simulink model "EvReferenceApplication"  (R2017b)
settings: Solver=ode23tb  StartTime=0  StopTime=600  RelTol=1e-3  EnableMultiTasking=on
InitFcn:
  | %open_system('EvReferenceApplication/Visualization/Performance and FE Scope');
undefined symbols (not defined in the file): ACC_Dgap_m, ACC_Kd, ACC_Ki, ACC_Kp, ACC_Nf, ACC_Tgap_s, BattChargeMax, UseAdaptiveCruiseControl_bool
libraries: autolibshared x2, autolibsharedcommon x1, simulink x1
settings Model: ModifiedByFormat=The MathWorks, Inc.  SimulationMode=accelerator  PauseTimes=23.46  Creator=The MathWorks, Inc.  LastModifiedBy=The MathWorks, Inc.
settings SolverCC: DecoupledContinuousIntegration=on
settings DataIOCC: DSMLogging=off
settings DebuggingCC: UnderspecifiedInitializationDetection=Classic  MergeDetectMultiDrivingBlocksExec=none  ModelReferenceExtraNoncontSigs=none
settings ModelReferenceCC: UpdateModelReferenceTargets=IfOutOfDate  EnableParallelModelReferenceBuilds=on  ModelReferenceMinAlgLoopOccurrences=on  PropagateSignalLabelsOutOfModel=off
settings CodeAppCC: StateflowObjectComments=on
settings GRTTargetCC: TargetLangStandard=C89/C90 (ANSI)
settings ConfigComp: CovMetricSettings=dsw  CovHtmlReporting=on  CovSaveCumulativeToWorkspaceVar=on  CovSaveSingleToWorkspaceVar=on  CovShowResultsExplorer=off  CovExternalEMLEnable=off

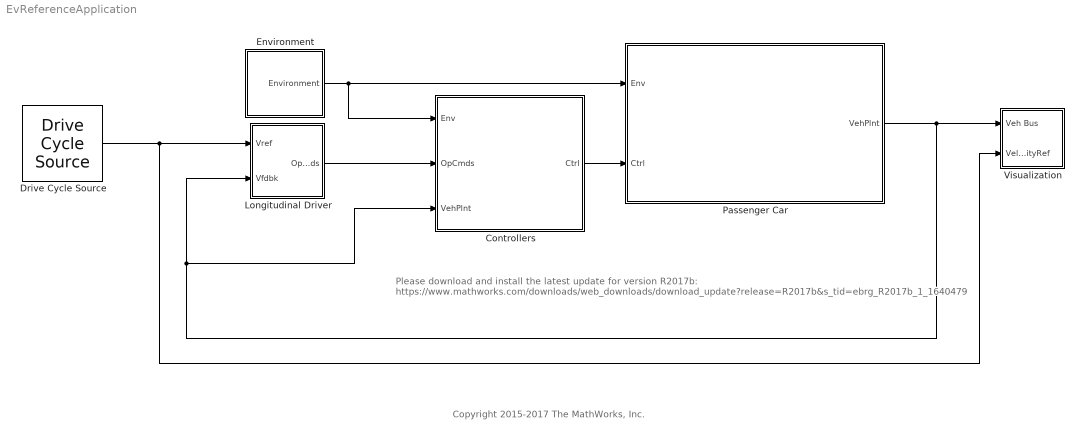
== system EvReferenceApplication ==
  note: Copyright 2015-2017 The MathWorks, Inc.
  note: Please download and install the latest update for version R2017b: https://www.mathworks.com/downloads/web_downloads/download_update?release=R2017b&s_tid=ebrg_R2017b_1_1640479
  Controllers : Subsystem
      mask Display: image('SystemControllers.png','center')
  Drive Cycle Source : autolibshared/Drive Cycle Source  cycleVar=US06  tfinal="600  seconds"  cycleRepeat=off  outAccPort=off  t_wot1=1  xdot_woto=0  xdot_wot1=26.8  t_wot2=30  xdot_wot2=0  t_wotend=40  srcUnit=m/s  outUnit=m/s  srcAccUnit=m/s/s  outAccUnit=m/s^2  dt=0
      settings: SourceProductName=Powertrain Blockset  SourceProductBaseCode=PW
  Environment : Subsystem
      mask Display: disp('Environment')
  Longitudinal Driver : Subsystem
      mask Display: image('LongitudinalDriver.png', 'center')
  Passenger Car : Subsystem
      mask Display: image('PassengerVehicle.png','center')
  Visualization : Subsystem
      mask Display: disp('Visualization')
  wires:
  Longitudinal Driver/1(OpCmds) -> Controllers/2(OpCmds)
  Drive Cycle Source/1 -> Longitudinal Driver/1(Vref), Visualization/2(VelocityRef)
  Environment/1(Environment) -> Controllers/1(Env), Passenger Car/1(Env)
  Controllers/1(Ctrl) -> Passenger Car/2(Ctrl)
  Passenger Car/1(VehPlnt) -> Controllers/3(VehPlnt), Longitudinal Driver/2(Vfdbk), Visualization/1(Veh Bus)

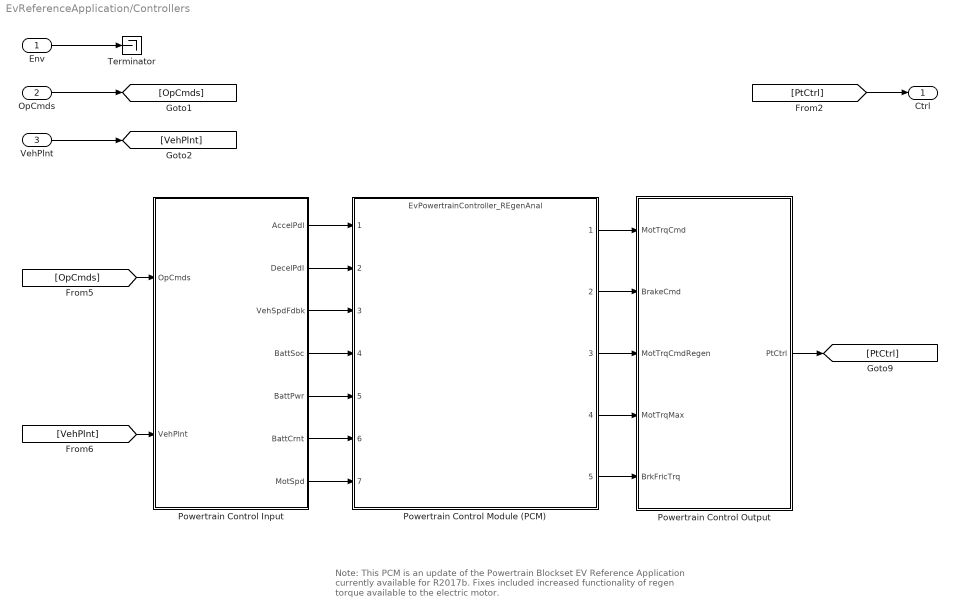
== system EvReferenceApplication/Controllers ==
  note: Note: This PCM is an update of the Powertrain Blockset EV Reference Application currently available for R2017b. Fixes included increased functionality of regen torque available to the electric motor.
  Env : Inport
  OpCmds : Inport  Port=2
  VehPlnt : Inport  Port=3
  Powertrain Control Input : Subsystem
  Powertrain Control Module (PCM) : ModelReference  ModelNameDialog=EvPowertrainController_REgenAnal.slx  SimulationMode=Normal  ModelReferenceVersion=1.420
  Powertrain Control Output : Subsystem
  Terminator : Terminator
  Ctrl : Outport
  wires:
  [PtCtrl] -> Ctrl/1
  Env/1 -> Terminator/1
  [OpCmds] -> Powertrain Control Input/1(OpCmds)
  Powertrain Control Output/1(PtCtrl) -> [PtCtrl]
  [VehPlnt] -> Powertrain Control Input/2(VehPlnt)
  VehPlnt/1 -> [VehPlnt]
  OpCmds/1 -> [OpCmds]
  Powertrain Control Input/4(BattSoc) -> Powertrain Control Module (PCM)/4
  Powertrain Control Input/3(VehSpdFdbk) -> Powertrain Control Module (PCM)/3
  Powertrain Control Input/2(DecelPdl) -> Powertrain Control Module (PCM)/2
  Powertrain Control Input/1(AccelPdl) -> Powertrain Control Module (PCM)/1
  Powertrain Control Input/5(BattPwr) -> Powertrain Control Module (PCM)/5
  Powertrain Control Input/6(BattCrnt) -> Powertrain Control Module (PCM)/6
  Powertrain Control Input/7(MotSpd) -> Powertrain Control Module (PCM)/7
  Powertrain Control Module (PCM)/1 -> Powertrain Control Output/1(MotTrqCmd)
  Powertrain Control Module (PCM)/2 -> Powertrain Control Output/2(BrakeCmd)
  Powertrain Control Module (PCM)/3 -> Powertrain Control Output/3(MotTrqCmdRegen)
  Powertrain Control Module (PCM)/4 -> Powertrain Control Output/4(MotTrqMax)
  Powertrain Control Module (PCM)/5 -> Powertrain Control Output/5(BrkFricTrq)

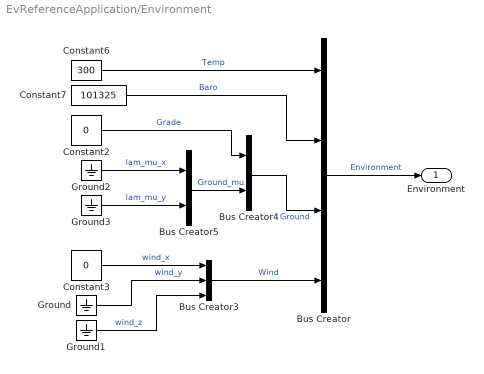
== system EvReferenceApplication/Environment ==
  Bus Creator : BusCreator  Inputs=4
  Bus Creator3 : BusCreator  Inputs=3
  Bus Creator4 : BusCreator  Inputs=2
  Bus Creator5 : BusCreator  Inputs=2
  Constant2 : Constant  Value=0
  Constant3 : Constant  Value=0
  Constant6 : Constant  Value=300
  Constant7 : Constant  Value=101325
  Ground{,1..3} (4 alike) : Ground
  Environment : Outport
  wires:
  Ground2/1 -> Bus Creator5/1  "lam_mu_x"
  Ground3/1 -> Bus Creator5/2  "lam_mu_y"
  Bus Creator5/1 -> Bus Creator4/2  "Ground_mu"
  Bus Creator4/1 -> Bus Creator/3  "Ground"
  Bus Creator3/1 -> Bus Creator/4  "Wind"
  Constant3/1 -> Bus Creator3/1  "wind_x"
  Ground/1 -> Bus Creator3/2  "wind_y"
  Ground1/1 -> Bus Creator3/3  "wind_z"
  Constant6/1 -> Bus Creator/1  "Temp"
  Constant2/1 -> Bus Creator4/1  "Grade"
  Bus Creator/1 -> Environment/1  "Environment"
  Constant7/1 -> Bus Creator/2  "Baro"

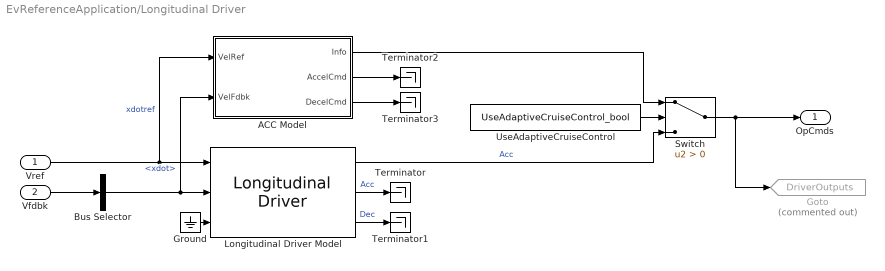
== system EvReferenceApplication/Longitudinal Driver ==
  Vref : Inport
  Vfdbk : Inport  Port=2
  ACC Model : Subsystem
  Bus Selector : BusSelector  OutputSignals=Veh.xdot
  Goto : Goto  Commented=on  GotoTag=DriverOutputs  TagVisibility=global
  Ground : Ground
  Longitudinal Driver Model : autolibshared/Longitudinal Driver  vnom=1  Kp=1  Ki=1  Kaw=1  Kff=0  Kg=0  tauerr=0
      settings: SourceProductName=Powertrain Blockset  SourceProductBaseCode=PW
  Switch : Switch  Criteria=u2 > Threshold
  Terminator{,1..3} (4 alike) : Terminator
  UseAdaptiveCruiseControl : Constant  Value=UseAdaptiveCruiseControl_bool  OutDataTypeStr=boolean
  OpCmds : Outport
  wires:
  UseAdaptiveCruiseControl/1 -> Switch/2
  Longitudinal Driver Model/1 -> Switch/3  "Acc"
  Switch/1 -> OpCmds/1, Goto/1
  ACC Model/1(Info) -> Switch/1
  ACC Model/3(DecelCmd) -> Terminator3/1
  ACC Model/2(AccelCmd) -> Terminator2/1
  Ground/1 -> Longitudinal Driver Model/3
  Longitudinal Driver Model/3 -> Terminator1/1  "Dec"
  Longitudinal Driver Model/2 -> Terminator/1  "Acc"
  Vfdbk/1 -> Bus Selector/1
  Vref/1 -> Longitudinal Driver Model/1, ACC Model/1(VelRef)  "xdotref"
  Bus Selector/1 -> Longitudinal Driver Model/2, ACC Model/2(VelFdbk)  "<xdot>"

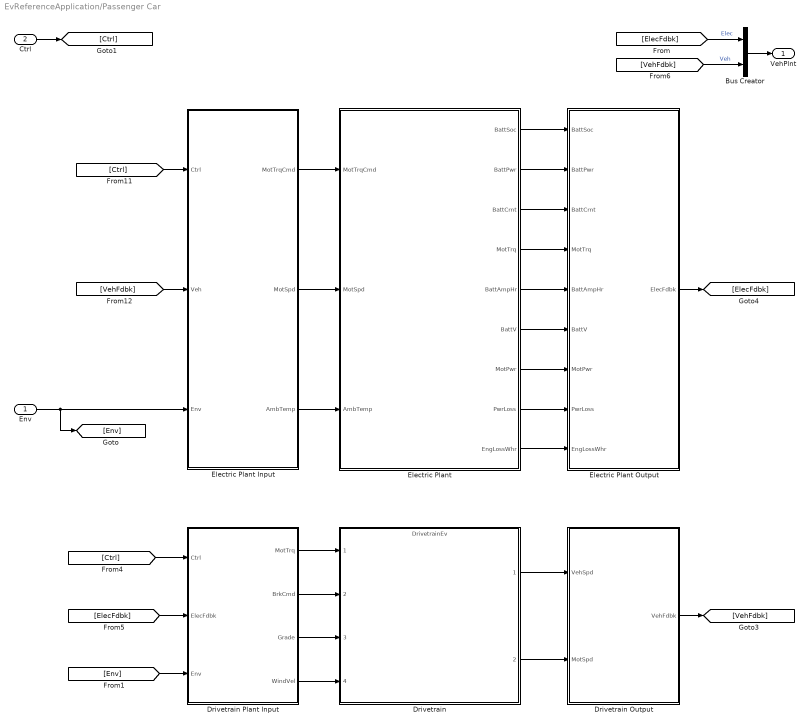
== system EvReferenceApplication/Passenger Car ==
  Env : Inport
  Ctrl : Inport  Port=2
  Bus Creator : BusCreator  Inputs=2
  Drivetrain : ModelReference  ModelNameDialog=DrivetrainEv.slx  SimulationMode=Normal  ModelReferenceVersion=1.424
  Drivetrain Output : Subsystem
  Drivetrain Plant Input : Subsystem
  Electric Plant : Subsystem
  Electric Plant Input : Subsystem
  Electric Plant Output : Subsystem
  VehPlnt : Outport
  wires:
  Drivetrain Plant Input/4(WindVel) -> Drivetrain/4
  Drivetrain Plant Input/3(Grade) -> Drivetrain/3
  [Env] -> Drivetrain Plant Input/3(Env)
  Electric Plant Input/3(AmbTemp) -> Electric Plant/3(AmbTemp)
  Electric Plant/4(MotTrq) -> Electric Plant Output/4(MotTrq)
  Electric Plant/3(BattCrnt) -> Electric Plant Output/3(BattCrnt)
  Electric Plant/2(BattPwr) -> Electric Plant Output/2(BattPwr)
  Electric Plant/1(BattSoc) -> Electric Plant Output/1(BattSoc)
  Electric Plant Input/2(MotSpd) -> Electric Plant/2(MotSpd)
  Electric Plant Input/1(MotTrqCmd) -> Electric Plant/1(MotTrqCmd)
  Drivetrain/1 -> Drivetrain Output/1(VehSpd)
  Drivetrain/2 -> Drivetrain Output/2(MotSpd)
  Drivetrain Plant Input/1(MotTrq) -> Drivetrain/1
  Drivetrain Plant Input/2(BrkCmd) -> Drivetrain/2
  [VehFdbk] -> Electric Plant Input/2(Veh)
  [ElecFdbk] -> Drivetrain Plant Input/2(ElecFdbk)
  [Ctrl] -> Electric Plant Input/1(Ctrl)
  [ElecFdbk] -> Bus Creator/1  "Elec"
  Electric Plant Output/1(ElecFdbk) -> [ElecFdbk]
  Drivetrain Output/1(VehFdbk) -> [VehFdbk]
  [VehFdbk] -> Bus Creator/2  "Veh"
  Bus Creator/1 -> VehPlnt/1
  [Ctrl] -> Drivetrain Plant Input/1(Ctrl)
  Env/1 -> Electric Plant Input/3(Env), [Env]
  Ctrl/1 -> [Ctrl]
  Electric Plant/5(BattAmpHr) -> Electric Plant Output/5(BattAmpHr)
  Electric Plant/6(BattV) -> Electric Plant Output/6(BattV)
  Electric Plant/7(MotPwr) -> Electric Plant Output/7(MotPwr)
  Electric Plant/8(PwrLoss) -> Electric Plant Output/8(PwrLoss)
  Electric Plant/9(EngLossWhr) -> Electric Plant Output/9(EngLossWhr)

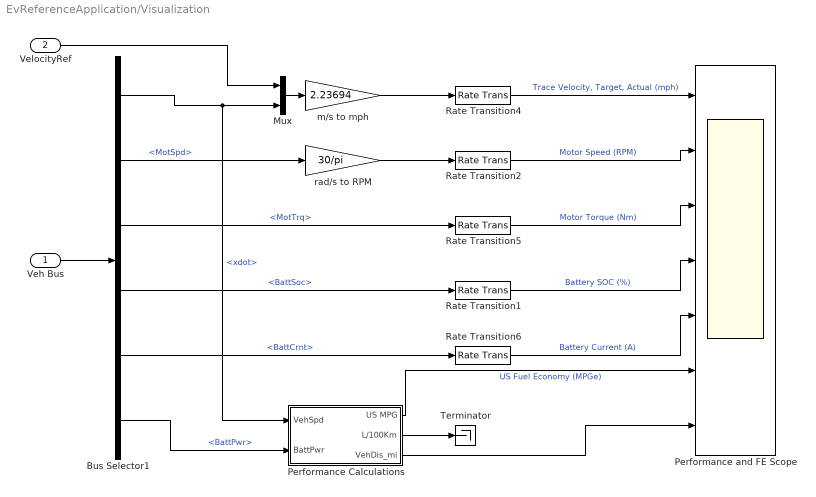
== system EvReferenceApplication/Visualization ==
  Veh Bus : Inport
  VelocityRef : Inport  Port=2
  Bus Selector1 : BusSelector  OutputSignals=Veh.xdot,Veh.MotSpd,Elec.MotTrq,Elec.BattSoc,Elec.BattCrnt,Elec.BattPwr
  Mux : Mux  Inputs=2
  Performance Calculations : Subsystem
  Performance and FE Scope : Scope  NumInputPorts=7
  Rate Transition{1..2,4..6} (5 alike) : RateTransition
  Terminator : Terminator
  m/s to mph : Gain  Gain=2.23694
  rad/s to RPM : Gain  Gain=30/pi
  wires:
  Veh Bus/1 -> Bus Selector1/1
  Bus Selector1/1 -> Performance Calculations/1(VehSpd), Mux/2  "<xdot>"
  Mux/1 -> m/s to mph/1
  Performance Calculations/1(US MPG) -> Performance and FE Scope/6  "US Fuel Economy (MPGe)"
  Performance Calculations/2(L/100Km) -> Terminator/1
  m/s to mph/1 -> Rate Transition4/1
  Bus Selector1/4 -> Rate Transition1/1  "<BattSoc>"
  VelocityRef/1 -> Mux/1
  Rate Transition1/1 -> Performance and FE Scope/4  "Battery SOC (%)"
  Rate Transition2/1 -> Performance and FE Scope/2  "Motor Speed (RPM)"
  Rate Transition4/1 -> Performance and FE Scope/1  "Trace Velocity, Target, Actual (mph)"
  Bus Selector1/2 -> rad/s to RPM/1  "<MotSpd>"
  Bus Selector1/6 -> Performance Calculations/2(BattPwr)  "<BattPwr>"
  rad/s to RPM/1 -> Rate Transition2/1
  Bus Selector1/3 -> Rate Transition5/1  "<MotTrq>"
  Rate Transition5/1 -> Performance and FE Scope/3  "Motor Torque (Nm)"
  Rate Transition6/1 -> Performance and FE Scope/5  "Battery Current (A)"
  Bus Selector1/5 -> Rate Transition6/1  "<BattCrnt>"
  Performance Calculations/3(VehDis_mi) -> Performance and FE Scope/7

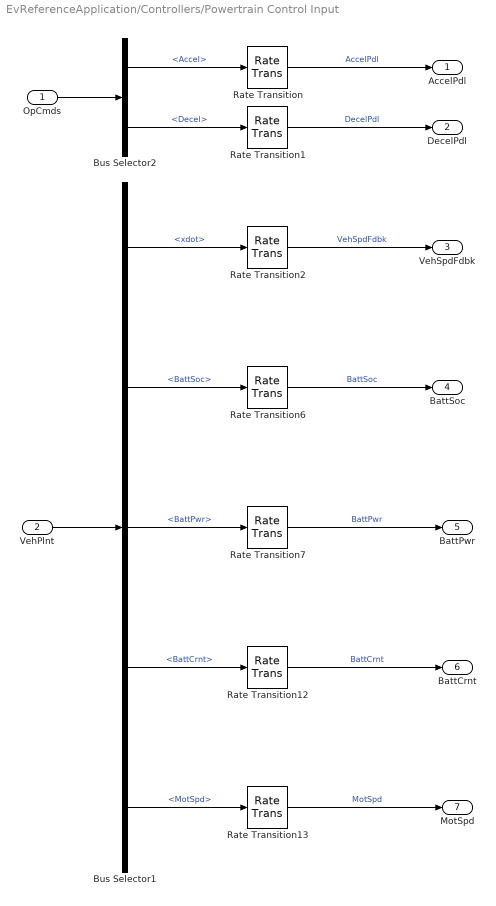
== system EvReferenceApplication/Controllers/Powertrain Control Input ==
  OpCmds : Inport
  VehPlnt : Inport  Port=2
  Bus Selector1 : BusSelector  OutputSignals=Veh.xdot,Elec.BattSoc,Elec.BattPwr,Elec.BattCrnt,Veh.MotSpd
  Bus Selector2 : BusSelector  OutputSignals=Accel,Decel
  Rate Transition{,1..2,6..7,12..13} (7 alike) : RateTransition  Deterministic=off
  AccelPdl : Outport
  DecelPdl : Outport  Port=2
  VehSpdFdbk : Outport  Port=3
  BattSoc : Outport  Port=4
  BattPwr : Outport  Port=5
  BattCrnt : Outport  Port=6
  MotSpd : Outport  Port=7
  wires:
  Bus Selector2/1 -> Rate Transition/1  "<Accel>"
  Rate Transition/1 -> AccelPdl/1  "AccelPdl"
  OpCmds/1 -> Bus Selector2/1
  Bus Selector2/2 -> Rate Transition1/1  "<Decel>"
  Rate Transition1/1 -> DecelPdl/1  "DecelPdl"
  Rate Transition2/1 -> VehSpdFdbk/1  "VehSpdFdbk"
  VehPlnt/1 -> Bus Selector1/1
  Rate Transition6/1 -> BattSoc/1  "BattSoc"
  Rate Transition7/1 -> BattPwr/1  "BattPwr"
  Rate Transition12/1 -> BattCrnt/1  "BattCrnt"
  Bus Selector1/1 -> Rate Transition2/1  "<xdot>"
  Bus Selector1/2 -> Rate Transition6/1  "<BattSoc>"
  Bus Selector1/3 -> Rate Transition7/1  "<BattPwr>"
  Bus Selector1/4 -> Rate Transition12/1  "<BattCrnt>"
  Rate Transition13/1 -> MotSpd/1  "MotSpd"
  Bus Selector1/5 -> Rate Transition13/1  "<MotSpd>"

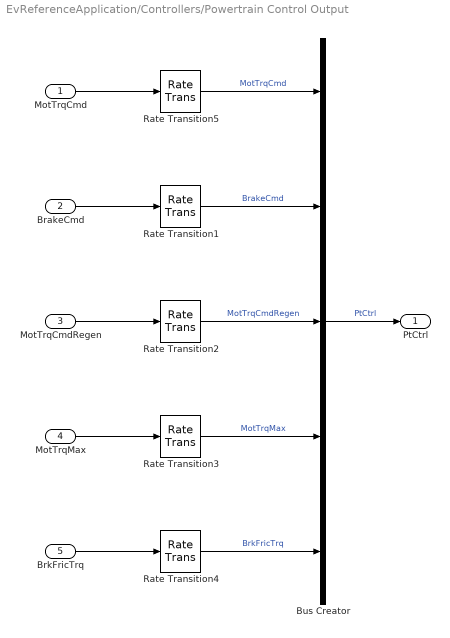
== system EvReferenceApplication/Controllers/Powertrain Control Output ==
  MotTrqCmd : Inport
  BrakeCmd : Inport  Port=2
  MotTrqCmdRegen : Inport  Port=3
  MotTrqMax : Inport  Port=4
  BrkFricTrq : Inport  Port=5
  Bus Creator : BusCreator  Inputs=5
  Rate Transition{1..5} (5 alike) : RateTransition  Deterministic=off
  PtCtrl : Outport
  wires:
  Rate Transition1/1 -> Bus Creator/2  "BrakeCmd"
  BrakeCmd/1 -> Rate Transition1/1
  Bus Creator/1 -> PtCtrl/1  "PtCtrl"
  Rate Transition5/1 -> Bus Creator/1  "MotTrqCmd"
  MotTrqCmd/1 -> Rate Transition5/1
  MotTrqCmdRegen/1 -> Rate Transition2/1
  Rate Transition2/1 -> Bus Creator/3  "MotTrqCmdRegen"
  MotTrqMax/1 -> Rate Transition3/1
  BrkFricTrq/1 -> Rate Transition4/1
  Rate Transition3/1 -> Bus Creator/4  "MotTrqMax"
  Rate Transition4/1 -> Bus Creator/5  "BrkFricTrq"

== system EvReferenceApplication/Longitudinal Driver/ACC Model ==
  VelRef : Inport
  VelFdbk : Inport  Port=2
  ACC Classical : Subsystem  TreatAsAtomicUnit=on  VariantControl=controller_type == 1
      settings: RTWFileNameOpts=Use function name
  HostPerceptionModel : Subsystem
  Info : Outport  InitialOutput=0
  AccelCmd : Outport  Port=2
  DecelCmd : Outport  Port=3
  wires:
  ACC Classical/3(DecelCmd) -> DecelCmd/1
  ACC Classical/1(Info) -> Info/1
  ACC Classical/2(AccelCmd) -> AccelCmd/1
  HostPerceptionModel/3(TargetRelSpd) -> ACC Classical/4(TargetRelSpd)
  HostPerceptionModel/1(EgoSpd) -> ACC Classical/2(EgoSpd)
  HostPerceptionModel/2(TargetRelPos) -> ACC Classical/3(TargetRelPos)
  VelFdbk/1 -> HostPerceptionModel/2(VelFdbk)
  VelRef/1 -> HostPerceptionModel/1(VelRef), ACC Classical/1(VelRef)

== system EvReferenceApplication/Passenger Car/Drivetrain Output ==
  VehSpd : Inport
  MotSpd : Inport  Port=2
  Bus Creator1 : BusCreator  Inputs=2
  VehFdbk : Outport
  wires:
  MotSpd/1 -> Bus Creator1/2  "MotSpd"
  VehSpd/1 -> Bus Creator1/1
  Bus Creator1/1 -> VehFdbk/1  "VehFdbk"

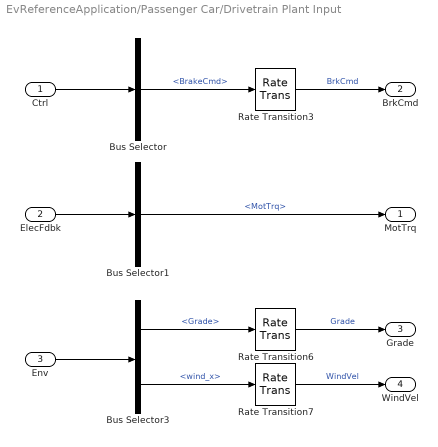
== system EvReferenceApplication/Passenger Car/Drivetrain Plant Input ==
  Ctrl : Inport
  ElecFdbk : Inport  Port=2
  Env : Inport  Port=3
  Bus Selector : BusSelector  OutputSignals=BrakeCmd
  Bus Selector1 : BusSelector  OutputSignals=MotTrq
  Bus Selector3 : BusSelector  OutputSignals=Ground.Grade,Wind.wind_x
  Rate Transition3 : RateTransition  Deterministic=off
  Rate Transition6 : RateTransition  Deterministic=off
  Rate Transition7 : RateTransition  Deterministic=off
  MotTrq : Outport
  BrkCmd : Outport  Port=2
  Grade : Outport  Port=3
  WindVel : Outport  Port=4
  wires:
  Bus Selector3/2 -> Rate Transition7/1  "<wind_x>"
  Bus Selector3/1 -> Rate Transition6/1  "<Grade>"
  Rate Transition7/1 -> WindVel/1  "WindVel"
  Rate Transition6/1 -> Grade/1  "Grade"
  Env/1 -> Bus Selector3/1
  Bus Selector1/1 -> MotTrq/1  "<MotTrq>"
  ElecFdbk/1 -> Bus Selector1/1
  Rate Transition3/1 -> BrkCmd/1  "BrkCmd"
  Bus Selector/1 -> Rate Transition3/1  "<BrakeCmd>"
  Ctrl/1 -> Bus Selector/1

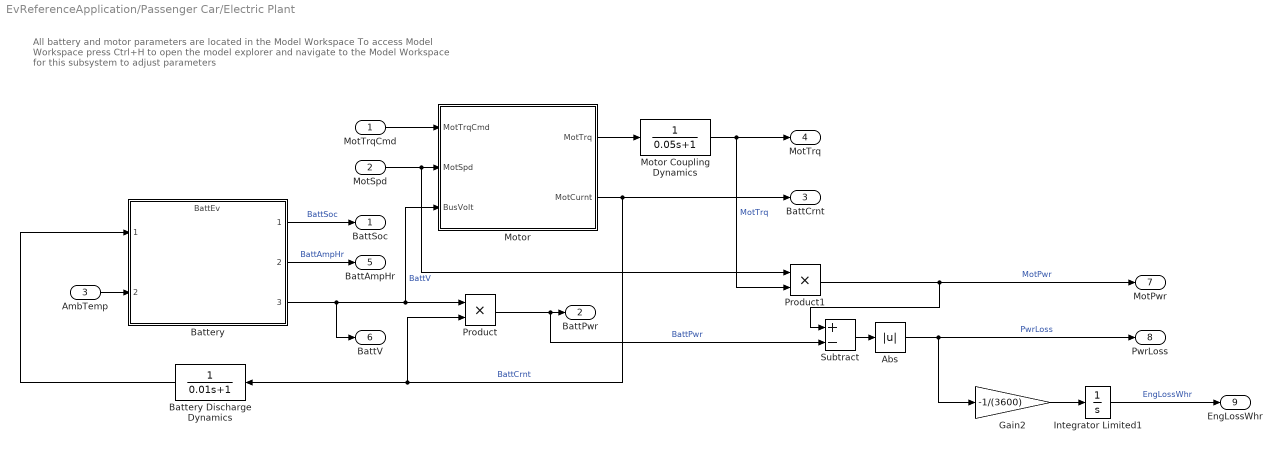
== system EvReferenceApplication/Passenger Car/Electric Plant ==
  note: All battery and motor parameters are located in the Model Workspace
      | To access Model Workspace press Ctrl+H to open the model explorer and navigate to the Model Workspace for this subsystem to adjust parameters
  MotTrqCmd : Inport
  MotSpd : Inport  Port=2
  AmbTemp : Inport  Port=3
  Abs : Abs
  Battery : ModelReference  ModelNameDialog=BattEv.slx  SimulationMode=Normal  ModelReferenceVersion=1.356
  Battery Discharge Dynamics : TransferFcn  Denominator=[0.01 1]
  Gain2 : Gain  Gain=-1/(3600)
  Integrator Limited1 : Integrator  UpperSaturationLimit=BattChargeMax  LowerSaturationLimit=0
  Motor : Subsystem  Variant=on  OverrideUsingVariant=MotGenEvMapped
  Motor Coupling Dynamics : TransferFcn  Denominator=[0.05 1]
  Product : Product
  Product1 : Product
  Subtract : Sum  Inputs=+-
  BattSoc : Outport
  BattPwr : Outport  Port=2
  BattCrnt : Outport  Port=3
  MotTrq : Outport  Port=4
  BattAmpHr : Outport  Port=5
  BattV : Outport  Port=6
  MotPwr : Outport  Port=7
  PwrLoss : Outport  Port=8
  EngLossWhr : Outport  Port=9
  wires:
  Motor Coupling Dynamics/1 -> Product1/2, MotTrq/1  "MotTrq"
  Battery Discharge Dynamics/1 -> Battery/1
  Motor/2(MotCurnt) -> BattCrnt/1, Product/2, Battery Discharge Dynamics/1  "BattCrnt"
  Product/1 -> Subtract/2, BattPwr/1  "BattPwr"
  Battery/3 -> BattV/1, Motor/3(BusVolt), Product/1  "BattV"
  Battery/1 -> BattSoc/1  "BattSoc"
  Motor/1(MotTrq) -> Motor Coupling Dynamics/1
  AmbTemp/1 -> Battery/2
  MotSpd/1 -> Product1/1, Motor/2(MotSpd)
  MotTrqCmd/1 -> Motor/1(MotTrqCmd)
  Battery/2 -> BattAmpHr/1  "BattAmpHr"
  Product1/1 -> Subtract/1, MotPwr/1  "MotPwr"
  Abs/1 -> Gain2/1, PwrLoss/1  "PwrLoss"
  Subtract/1 -> Abs/1
  Gain2/1 -> Integrator Limited1/1
  Integrator Limited1/1 -> EngLossWhr/1  "EngLossWhr"

== system EvReferenceApplication/Passenger Car/Electric Plant Input ==
  Ctrl : Inport
  Veh : Inport  Port=2
  Env : Inport  Port=3
  Bus Selector : BusSelector  OutputSignals=MotTrqCmd
  Bus Selector1 : BusSelector  OutputSignals=MotSpd
  Bus Selector2 : BusSelector  OutputSignals=Temp
  Rate Transition1 : RateTransition  Deterministic=off
  Rate Transition5 : RateTransition  Deterministic=off
  MotTrqCmd : Outport
  MotSpd : Outport  Port=2
  AmbTemp : Outport  Port=3
  wires:
  Bus Selector2/1 -> Rate Transition1/1  "<Temp>"
  Rate Transition1/1 -> AmbTemp/1  "AmbTmp"
  Env/1 -> Bus Selector2/1
  Bus Selector1/1 -> MotSpd/1  "<MotSpd>"
  Veh/1 -> Bus Selector1/1
  Bus Selector/1 -> Rate Transition5/1  "<MotTrqCmd>"
  Ctrl/1 -> Bus Selector/1
  Rate Transition5/1 -> MotTrqCmd/1  "MotTrqCmd"

== system EvReferenceApplication/Passenger Car/Electric Plant Output ==
  BattSoc : Inport
  BattPwr : Inport  Port=2
  BattCrnt : Inport  Port=3
  MotTrq : Inport  Port=4
  BattAmpHr : Inport  Port=5
  BattV : Inport  Port=6
  MotPwr : Inport  Port=7
  PwrLoss : Inport  Port=8
  EngLossWhr : Inport  Port=9
  Bus Creator1 : BusCreator  Inputs=9
  ElecFdbk : Outport
  wires:
  MotTrq/1 -> Bus Creator1/4
  BattCrnt/1 -> Bus Creator1/3
  BattSoc/1 -> Bus Creator1/1
  BattPwr/1 -> Bus Creator1/2
  Bus Creator1/1 -> ElecFdbk/1  "ElecFdbk"
  BattAmpHr/1 -> Bus Creator1/5
  BattV/1 -> Bus Creator1/6
  MotPwr/1 -> Bus Creator1/7
  PwrLoss/1 -> Bus Creator1/8
  EngLossWhr/1 -> Bus Creator1/9

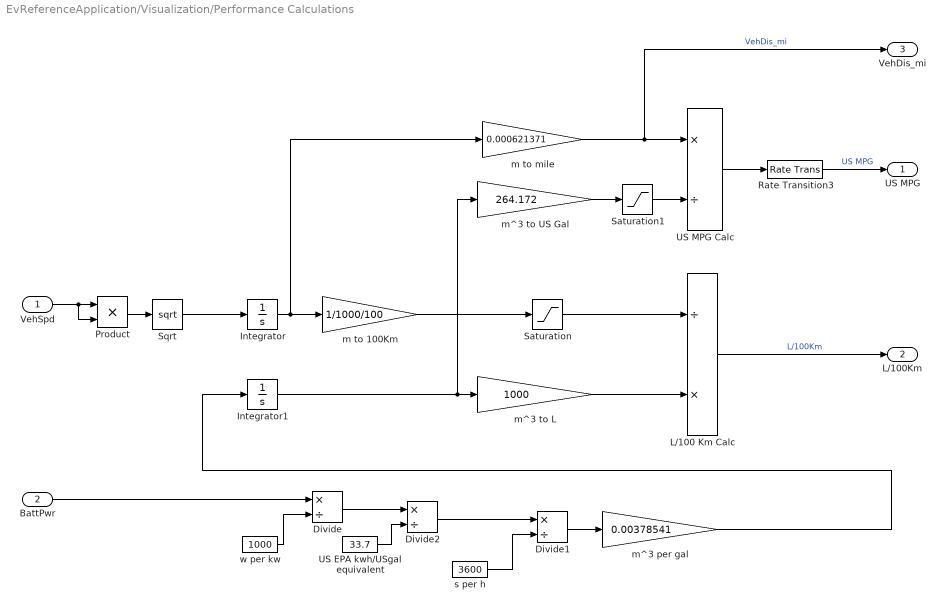
== system EvReferenceApplication/Visualization/Performance Calculations ==
  VehSpd : Inport
  BattPwr : Inport  Port=2
  Divide : Product  Inputs=*/
  Divide1 : Product  Inputs=*/
  Divide2 : Product  Inputs=*/
  Integrator : Integrator
  Integrator1 : Integrator
  L/100 Km Calc : Product  Inputs=/*
  Product : Product
  Rate Transition3 : RateTransition
  Saturation : Saturate  UpperLimit=Inf  LowerLimit=0.1
  Saturation1 : Saturate  UpperLimit=Inf  LowerLimit=1e-3
  Sqrt : Sqrt  SaturateOnIntegerOverflow=on
  US EPA kwh/USgal equivalent : Constant  Value=33.7
  US MPG Calc : Product  Inputs=*/
  m to 100Km : Gain  Gain=1/1000/100
  m to mile : Gain  Gain=0.000621371
  m^3 per gal : Gain  Gain=0.00378541
  m^3 to L : Gain  Gain=1000
  m^3 to US Gal : Gain  Gain=264.172
  s per h : Constant  Value=3600
  w per kw : Constant  Value=1000
  US MPG : Outport
  L/100Km : Outport  Port=2
  VehDis_mi : Outport  Port=3
  wires:
  m^3 to US Gal/1 -> Saturation1/1
  m^3 to L/1 -> L/100 Km Calc/2
  Integrator/1 -> m to mile/1, m to 100Km/1
  m to mile/1 -> VehDis_mi/1, US MPG Calc/1  "VehDis_mi"
  Integrator1/1 -> m^3 to US Gal/1, m^3 to L/1
  Saturation/1 -> L/100 Km Calc/1
  m to 100Km/1 -> Saturation/1
  L/100 Km Calc/1 -> L/100Km/1  "L/100Km"
  US MPG Calc/1 -> Rate Transition3/1
  Saturation1/1 -> US MPG Calc/2
  Rate Transition3/1 -> US MPG/1  "US MPG"
  w per kw/1 -> Divide/2
  Divide/1 -> Divide2/1
  Divide2/1 -> Divide1/1
  s per h/1 -> Divide1/2
  Divide1/1 -> m^3 per gal/1
  m^3 per gal/1 -> Integrator1/1
  US EPA kwh/USgal equivalent/1 -> Divide2/2
  BattPwr/1 -> Divide/1
  Sqrt/1 -> Integrator/1
  Product/1 -> Sqrt/1
  VehSpd/1 -> Product/2, Product/1

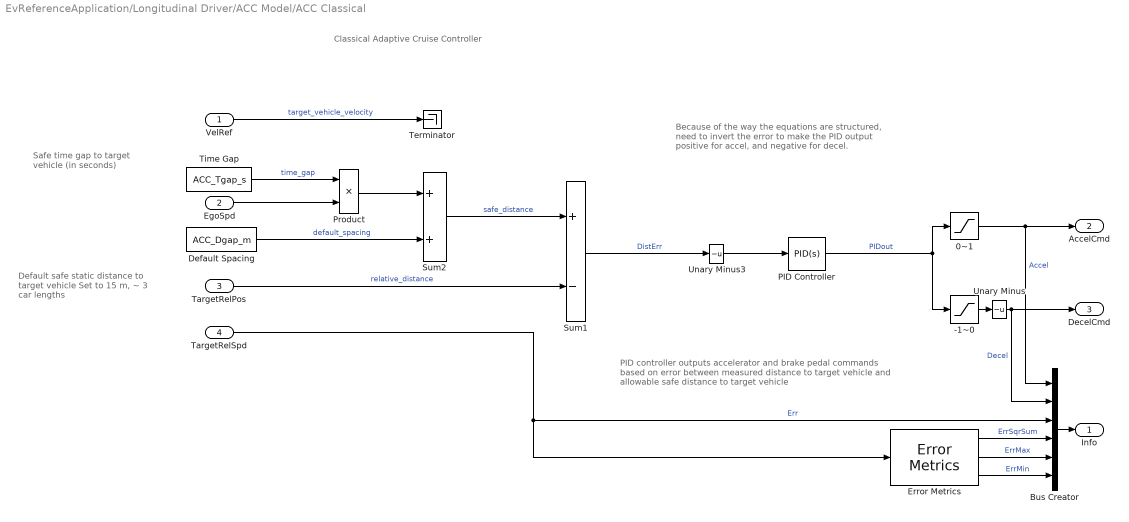
== system EvReferenceApplication/Longitudinal Driver/ACC Model/ACC Classical ==
  note: Classical Adaptive Cruise Controller
  note: Default safe static distance to target vehicle
      | Set to 15 m, ~ 3 car lengths
  note: PID controller outputs accelerator and brake pedal commands based on error between measured distance to target vehicle and allowable safe distance to target vehicle
  note: Because of the way the equations are structured,
      | need to invert the error to make the PID output
      | positive for accel, and negative for decel.
  note: Safe time gap to target vehicle (in seconds)
  VelRef : Inport
  EgoSpd : Inport  Port=2
  TargetRelPos : Inport  Port=3
  TargetRelSpd : Inport  Port=4
  -1~0 : Saturate  UpperLimit=0  LowerLimit=-1  ZeroCross=off
  0~1 : Saturate  UpperLimit=1  LowerLimit=0  ZeroCross=off
  Bus Creator : BusCreator  Inputs=6
  Default Spacing : Constant  Value=ACC_Dgap_m  SampleTime=-1
  Error Metrics : autolibsharedcommon/Longitudinal Driver/Error Metrics
      settings: SourceProductName=Powertrain Blockset  SourceProductBaseCode=PW
  PID Controller : simulink/Continuous/PID Controller  Controller=PID  TimeDomain=Continuous-time  SampleTime=-1  IntegratorMethod=Forward Euler  FilterMethod=Forward Euler  Form=Parallel  UseFilter=on  ControllerParametersSource=internal  P=ACC_Kp  I=ACC_Ki  D=ACC_Kd  N=ACC_Nf  InitialConditionSource=internal  InitialConditionForIntegrator=0  InitialConditionForFilter=0  ExternalReset=none  LimitOutput=on  UpperSaturationLimit=1  LowerSaturationLimit=-1  LinearizeAsGain=on  AntiWindupMode=clamping  Kb=1  TrackingMode=off  Kt=1  PParamMin=[]  PParamMax=[]  IParamMin=[]  IParamMax=[]  DParamMin=[]  DParamMax=[]  NParamMin=[]  NParamMax=[]  KbParamMin=[]  KbParamMax=[]  KtParamMin=[]  KtParamMax=[]  POutMin=[]  POutMax=[]  IOutMin=[]  IOutMax=[]  DOutMin=[]  DOutMax=[]  NOutMin=[]  NOutMax=[]  KbOutMin=[]  KbOutMax=[]  KtOutMin=[]  KtOutMax=[]  IntegratorOutMin=[]  IntegratorOutMax=[]  FilterOutMin=[]  FilterOutMax=[]  SumOutMin=[]  SumOutMax=[]  SumI1OutMin=[]  SumI1OutMax=[]  SumI2OutMin=[]  SumI2OutMax=[]  SumI3OutMin=[]  SumI3OutMax=[]  SumDOutMin=[]  SumDOutMax=[]  SaturationOutMin=[]  SaturationOutMax=[]  IntegratorContinuousStateAttributes=''  IntegratorStateMustResolveToSignalObject=off  IntegratorRTWStateStorageClass=Auto  FilterContinuousStateAttributes=''  FilterStateMustResolveToSignalObject=off  FilterRTWStateStorageClass=Auto  DifferentiatorICPrevScaledInput=0  DifferentiatorOutMin=[]  DifferentiatorOutMax=[]  InitialConditionSetting=State (most efficient)  FilterDiffOutCoefMin=[]  FilterDiffOutCoefMax=[]  SumDenOutMin=[]  SumDenOutMax=[]  SumNumOutMin=[]  SumNumOutMax=[]  ReciprocalOutMin=[]  ReciprocalOutMax=[]  DivideOutMin=[]  DivideOutMax=[]  TunerSelectOption=Transfer Function Based (PID Tuner App)
  Product : Product
  Sum1 : Sum  Inputs=+-
  Sum2 : Sum
  Terminator : Terminator
  Time Gap : Constant  Value=ACC_Tgap_s  SampleTime=-1
  Unary Minus : UnaryMinus
  Unary Minus3 : UnaryMinus
  Info : Outport  InitialOutput=0
  AccelCmd : Outport  Port=2  Unit=one  InitialOutput=0
  DecelCmd : Outport  Port=3  Unit=one  InitialOutput=0
  wires:
  EgoSpd/1 -> Product/2
  Unary Minus3/1 -> PID Controller/1
  Error Metrics/1 -> Bus Creator/4  "ErrSqrSum"
  Error Metrics/2 -> Bus Creator/5  "ErrMax"
  Bus Creator/1 -> Info/1
  Error Metrics/3 -> Bus Creator/6  "ErrMin"
  -1~0/1 -> Unary Minus/1
  Unary Minus/1 -> Bus Creator/2, DecelCmd/1  "Decel"
  PID Controller/1 -> -1~0/1, 0~1/1  "PIDout"
  0~1/1 -> AccelCmd/1, Bus Creator/1  "Accel"
  TargetRelPos/1 -> Sum1/2  "relative_distance"
  Sum1/1 -> Unary Minus3/1  "DistErr"
  VelRef/1 -> Terminator/1  "target_vehicle_velocity"
  Sum2/1 -> Sum1/1  "safe_distance"
  Product/1 -> Sum2/1
  Time Gap/1 -> Product/1  "time_gap"
  TargetRelSpd/1 -> Bus Creator/3, Error Metrics/1  "Err"
  Default Spacing/1 -> Sum2/2  "default_spacing"

== system EvReferenceApplication/Longitudinal Driver/ACC Model/HostPerceptionModel ==
  VelRef : Inport
  VelFdbk : Inport  Port=2
  Add : Sum  Inputs=+-+
  Add1 : Sum  Inputs=+-
  Data Type Conversion : DataTypeConversion
  Integrator : Integrator
  Integrator1 : Integrator
  TargetInitialPos : Constant  Value=15
  EgoSpd : Outport
  TargetRelPos : Outport  Port=2
  TargetRelSpd : Outport  Port=3
  wires:
  VelFdbk/1 -> Integrator/1, Data Type Conversion/1, Add1/2
  Integrator1/1 -> Add/1  "TargetPos"
  Integrator/1 -> Add/2  "EgoPos"
  Add/1 -> TargetRelPos/1  "TargetRelPos"
  Data Type Conversion/1 -> EgoSpd/1  "EgoSpd"
  Add1/1 -> TargetRelSpd/1  "TargetRelSpd"
  TargetInitialPos/1 -> Add/3
  VelRef/1 -> Add1/1, Integrator1/1

== system EvReferenceApplication/Passenger Car/Electric Plant/Motor ==
  MotTrqCmd : Inport
  MotSpd : Inport  Port=2
  BusVolt : Inport  Port=3
  MotGenEvDynamic : ModelReference  ModelNameDialog=MotGenEvDynamic.slx  SimulationMode=Normal  VariantControl=MotGenEvDynamic  ModelReferenceVersion=1.347
  MotGenEvMapped : ModelReference  ModelNameDialog=MotGenEvMapped.slx  SimulationMode=Normal  VariantControl=MotGenEvMapped  ModelReferenceVersion=1.357
  MotTrq : Outport
  MotCurnt : Outport  Port=2
